simulink model "Ex72"  (R2019a)
settings: Solver=VariableStepAuto  StartTime=0.0  StopTime=10.0  RelTol=1e-3
settings Model: Creator=toshi  LastModifiedBy=toshi

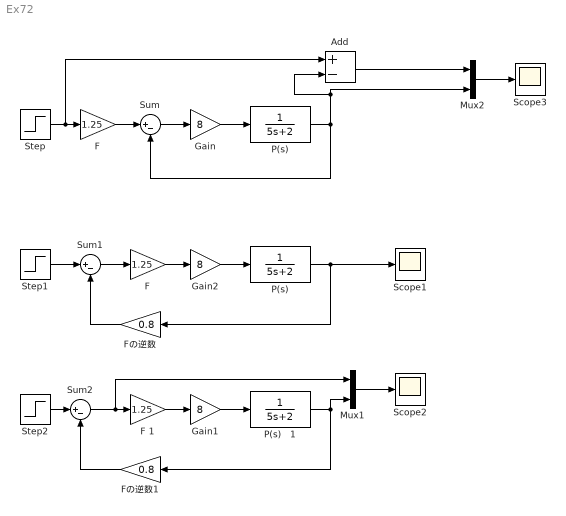
== system Ex72 ==
  Add : Sum  Inputs=+-
  F : Gain  Gain=1.25
  "F " : Gain  Gain=1.25
  F 1 : Gain  Gain=1.25
  Fの逆数 : Gain  Gain=0.8
  Fの逆数1 : Gain  Gain=0.8
  Gain : Gain  Gain=8
  Gain1 : Gain  Gain=8
  Gain2 : Gain  Gain=8
  Mux1 : Mux  Inputs=2
  Mux2 : Mux  Inputs=2
  P(s) : TransferFcn  Denominator=[5 2]
  "P(s)　" : TransferFcn  Denominator=[5 2]
  P(s)　1 : TransferFcn  Denominator=[5 2]
  Scope1 : Scope
  Scope2 : Scope
  Scope3 : Scope
  Step : Step  Time=0  SampleTime=0
  Step1 : Step  Time=0  SampleTime=0
  Step2 : Step  Time=0  SampleTime=0
  Sum : Sum  Inputs=|+-
  Sum1 : Sum  Inputs=|+-
  Sum2 : Sum  Inputs=|+-
  wires:
  Gain/1 -> P(s)/1
  P(s)/1 -> Add/2, Mux2/2, Sum/2
  Sum/1 -> Gain/1
  Step/1 -> Add/1, F/1
  F/1 -> Sum/1
  Gain2/1 -> "P(s)　"/1
  Sum1/1 -> "F "/1
  Step1/1 -> Sum1/1
  "F "/1 -> Gain2/1
  Fの逆数/1 -> Sum1/2
  "P(s)　"/1 -> Scope1/1, Fの逆数/1
  F 1/1 -> Gain1/1
  Step2/1 -> Sum2/1
  Sum2/1 -> Mux1/1, F 1/1
  Fの逆数1/1 -> Sum2/2
  Gain1/1 -> P(s)　1/1
  P(s)　1/1 -> Mux1/2, Fの逆数1/1
  Mux1/1 -> Scope2/1
  Mux2/1 -> Scope3/1
  Add/1 -> Mux2/1
